simulink model "solve_eqn"  (R2023a)
settings: Solver=VariableStepAuto  StartTime=0.0  StopTime=10.0  RelTol=1e-3
values from neighbouring files (symbols this model uses):
  damping = 5000    [Solving_Equation_of_Motion.m]    (also in Solving_Equation_with_simulink.m = 100; Solving_Equation_with_state_space_representation.m = 0)
  mass = 750    [Solving_Equation_of_Motion.m]    (also in Solving_Equation_with_simulink.m; Solving_Equation_with_state_space_representation.m; exercise1.m)
  stiffness = 1000000    [Solving_Equation_of_Motion.m]    (also in Solving_Equation_with_simulink.m = 5000; Solving_Equation_with_state_space_representation.m = 50000; exercise1.m = 50000)
  x_0 = 0.01    [Solving_Equation_of_Motion.m]    (also in Solving_Equation_with_simulink.m; Solving_Equation_with_state_space_representation.m; exercise1.m)
  x_dot_0 = 0.1    [Solving_Equation_of_Motion.m]    (also in Solving_Equation_with_simulink.m; Solving_Equation_with_state_space_representation.m = 0; exercise1.m = 0)
settings Model: Creator=Neeraj  LastModifiedBy=Neeraj

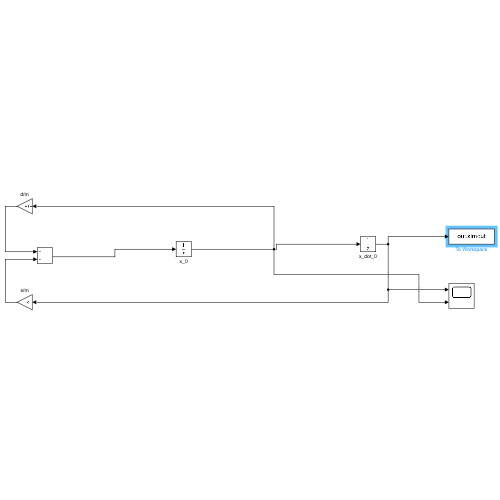
[thumbnail: Simulink's stored preview of the top-level diagram]
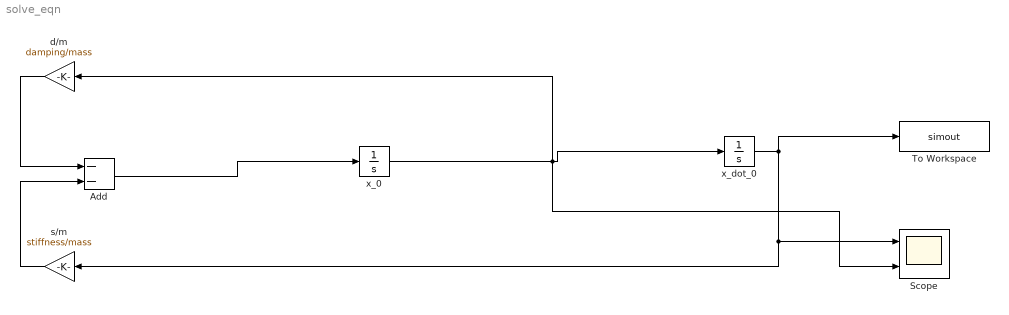
== system solve_eqn ==
  Add : Sum  Inputs=--
  Scope : Scope  NumInputPorts=2
  To Workspace : ToWorkspace  VariableName=simout  SaveFormat=Timeseries  SampleTime=-1
  d/m : Gain  Gain=damping/mass
  s/m : Gain  Gain=stiffness/mass
  x_0 : Integrator  InitialCondition=x_0
  x_dot_0 : Integrator  InitialCondition=x_dot_0
  wires:
  x_0/1 -> Scope/2, d/m/1, x_dot_0/1
  s/m/1 -> Add/2
  d/m/1 -> Add/1
  Add/1 -> x_0/1
  x_dot_0/1 -> To Workspace/1, Scope/1, s/m/1
